simulink model "omni_interface"  (Simulink 7.0)
settings: Solver=ode1  StartTime=0.0  StopTime=inf  FixedStep=0.001  RelTol=1e-3
undefined symbols (not defined in the file): HIL
libraries: quarc_library x8, simulink x7
settings Model: Creator=colinlea  LastModifiedBy=colinlea  SimulationMode=external  ExtModeTrigDuration=10000
settings SolverCC: PositivePriorityOrder=on
settings RTWCC: SystemTargetFile=quarc_windows.tlc  TemplateMakefile=quarc_default_tmf  Description=QuaRC Win32 Target  ProcessScript=quarc_windows_make_rtw_hook
settings STFCustomTargetCC: TargetPreCompLibLocation=C:\DOCUME~1\ALLUSE~1\APPLIC~1\QuaRC\lib\2007b\windows\release  GenFloatMathFcnCalls=ANSI_C  SystemTargetFile=quarc_windows.tlc
settings GRTTargetCC: TargetPreCompLibLocation=C:\DOCUME~1\ALLUSE~1\APPLIC~1\QuaRC\lib\2007b\windows\release  CompOptLevelCompliant=off  MatFileLogging=off  ExtMode=on  ExtModeMexFile=quarc_comm

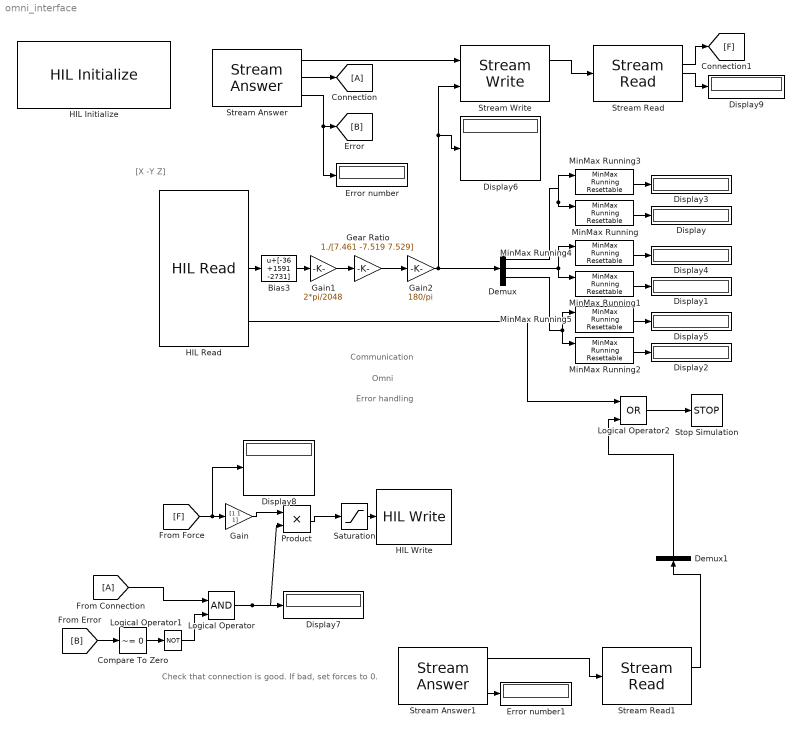
== system omni_interface ==
  note: [X -Y Z]
  note: Check that connection is good.
      | If bad, set forces to 0.
  note: Communication
  note: Omni
  note: Error handling
  Bias3 : Bias  Bias=[-36 +1591 -2731]
  Compare To Zero : simulink/Logic and Bit Operations/Compare To Zero  SystemSampleTime=-1  relop=~=  LogicOutDataTypeMode=uint8  ZeroCross=off
  Demux : Demux  Outputs=3
  Demux1 : Demux  Orientation=up  Outputs=3
  Display{,1..9} (10 alike) : Display
  Error number : Display
  Error number1 : Display
  Gain : Gain  Gain=[1 1 1]  ParameterDataType=sfix(16)  ParameterScaling=2^0  OutDataType=sfix(16)  OutScaling=2^0
  Gain1 : Gain  Gain=2*pi/2048  ParameterDataType=sfix(16)  ParameterScaling=2^0  OutDataType=sfix(16)  OutScaling=2^0
  Gain2 : Gain  Gain=180/pi  ParameterDataType=sfix(16)  ParameterScaling=2^0  OutDataType=sfix(16)  OutScaling=2^0
  Gear Ratio : Gain  Gain=1./[7.461 -7.519 7.529]  ParameterDataType=sfix(16)  ParameterScaling=2^0  OutDataType=sfix(16)  OutScaling=2^0
  HIL Initialize : quarc_library/Data Acquisition/Generic/Configuration/HIL Initialize  object_name=HIL-1  board_type=phantom_omni  board_number=0  active=on  hardware_clocks=[]  clock_modes=[]  set_clock_params_at_start=off  set_clock_params_at_switch_in=off  analog_input_channels=0:1  analog_input_maximums=10  analog_input_minimums=-10  set_analog_input_params_at_start=off  set_analog_input_params_at_switch_in=off  analog_output_channels=[]  analog_output_maximums=[]  analog_output_minimums=[]  initial_analog_outputs=[]  final_analog_outputs=[]  watchdog_analog_outputs=[]  set_analog_output_params_at_start=off  set_analog_output_params_at_switch_in=off  set_analog_outputs_at_start=off  set_analog_outputs_at_switch_in=off  set_analog_outputs_at_terminate=off  set_analog_outputs_at_switch_out=off  set_analog_outputs_on_watchdog=off  digital_input_channels=[]  digital_output_channels=[]  initial_digital_outputs=[]  final_digital_outputs=[]  watchdog_digital_outputs=[]  set_digital_outputs_at_start=off  set_digital_outputs_at_switch_in=off  set_digital_outputs_at_terminate=off  set_digital_outputs_at_switch_out=off  set_digital_outputs_on_watchdog=off  encoder_channels=0:2  quadrature=[]  encoder_filter_frequency=[]  initial_encoder_counts=0  set_encoder_params_at_start=off  set_encoder_params_at_switch_in=off  set_encoder_counts_at_start=off  set_encoder_counts_at_switch_in=off  pwm_channels=0:2  pwm_modes=[]  pwm_frequency=[]  initial_pwm_outputs=0  final_pwm_outputs=0  watchdog_pwm_outputs=[]  set_pwm_params_at_start=off  set_pwm_params_at_switch_in=off  set_pwm_outputs_at_start=on  set_pwm_outputs_at_switch_in=off  set_pwm_outputs_at_terminate=on  set_pwm_outputs_at_switch_out=off  set_pwm_outputs_on_watchdog=off  other_output_channels=[]  initial_other_outputs=[]  final_other_outputs=[]  watchdog_other_outputs=[]  set_other_outputs_at_start=off  set_other_outputs_at_switch_in=off  set_other_outputs_at_terminate=off  set_other_outputs_at_switch_out=off  set_other_outputs_on_watchdog=off
  HIL Read : quarc_library/Data Acquisition/Generic/Immediate I//O/HIL Read  object_name=HIL-1  analog_channels=[0:2]  encoder_channels=[0:2]  digital_channels=[0:1]  other_channels=[]  sample_time=qc_get_step_size  active=on  vector_output=on  data_type_mode=Inherit via back propagation  encoder_data_type=double  digital_data_type=boolean
  HIL Write : quarc_library/Data Acquisition/Generic/Immediate I//O/HIL Write  object_name=HIL-1  analog_channels=[]  pwm_channels=[0:2]  digital_channels=[]  other_channels=[]  sample_time=-1  active=off  vector_input=on
  Logical Operator : Logic  IconShape=distinctive  AllPortsSameDT=off  OutDataTypeMode=boolean
  Logical Operator1 : Logic  Operator=NOT  IconShape=distinctive  AllPortsSameDT=off  OutDataTypeMode=boolean
  Logical Operator2 : Logic  Operator=OR  Inputs=3  IconShape=distinctive  AllPortsSameDT=off  OutDataTypeMode=boolean
  MinMax Running : simulink/Math Operations/MinMax Running Resettable  SystemSampleTime=-1  Function=min  vinit=0.0
  MinMax Running1 : simulink/Math Operations/MinMax Running Resettable  SystemSampleTime=-1  Function=min  vinit=0.0
  MinMax Running2 : simulink/Math Operations/MinMax Running Resettable  SystemSampleTime=-1  Function=min  vinit=0.0
  MinMax Running3 : simulink/Math Operations/MinMax Running Resettable  SystemSampleTime=-1  Function=max  vinit=0.0
  MinMax Running4 : simulink/Math Operations/MinMax Running Resettable  SystemSampleTime=-1  Function=max  vinit=0.0
  MinMax Running5 : simulink/Math Operations/MinMax Running Resettable  SystemSampleTime=-1  Function=max  vinit=0.0
  Product : Product  OutDataType=sfix(16)  OutScaling=2^0  RndMeth=Zero
  Saturation : Saturate  UpperLimit=1  LowerLimit=-1  OutDataType=sfix(16)  OutScaling=2^0
  Stop Simulation : Stop
  Stream Answer : quarc_library/Communications/Intermediate/Stream Answer  uri_source=Internal (dialog parameter)  uri=tcpip://localhost:18000  send_buffer_size=8000  receive_buffer_size=8000  byte_order=little endian (Intel - LSB first)  sample_time=qc_get_step_size  active=off
      settings: AttributesFormatString=(%<uri>)
  Stream Answer1 : quarc_library/Communications/Intermediate/Stream Answer  uri_source=Internal (dialog parameter)  uri=tcpip://localhost:18002  send_buffer_size=8000  receive_buffer_size=8000  byte_order=little endian (Intel - LSB first)  sample_time=qc_get_step_size  active=off
      settings: AttributesFormatString=(%<uri>)
  Stream Read : quarc_library/Communications/Intermediate/Stream Read  data_type=Inherited via back propagation  num_elements=3
  Stream Read1 : quarc_library/Communications/Intermediate/Stream Read  data_type=Inherited via back propagation  num_elements=3
  Stream Write : quarc_library/Communications/Intermediate/Stream Write  optimization=Minimizing latency
  wires:
  Saturation/1 -> HIL Write/1
  MinMax Running/1 -> Display/1
  MinMax Running1/1 -> Display1/1
  MinMax Running2/1 -> Display2/1
  MinMax Running3/1 -> Display3/1
  MinMax Running4/1 -> Display4/1
  MinMax Running5/1 -> Display5/1
  Demux/1 -> MinMax Running/1, MinMax Running3/1
  Demux/2 -> MinMax Running1/1, MinMax Running4/1
  Demux/3 -> MinMax Running2/1, MinMax Running5/1
  HIL Read/2 -> Bias3/1
  Bias3/1 -> Gain1/1
  Gain1/1 -> Gear Ratio/1
  Gear Ratio/1 -> Gain2/1
  Stream Answer/1 -> Stream Write/1
  Gain2/1 -> Demux/1, Display6/1, Stream Write/2
  Gain/1 -> Product/1
  Product/1 -> Saturation/1
  Stream Answer/2 -> [A]
  Stream Answer/3 -> [B], Error number/1
  [B] -> Compare To Zero/1
  [A] -> Logical Operator/1
  Logical Operator/1 -> Product/2, Display7/1
  Stream Write/1 -> Stream Read/1
  Stream Read/2 -> [F]
  [F] -> Gain/1, Display8/1
  Stream Read/3 -> Display9/1
  Compare To Zero/1 -> Logical Operator1/1
  Logical Operator1/1 -> Logical Operator/2
  HIL Read/3 -> Logical Operator2/1
  Logical Operator2/1 -> Stop Simulation/1
  Stream Answer1/1 -> Stream Read1/1
  Stream Answer1/3 -> Error number1/1
  Stream Read1/2 -> Demux1/1
  Demux1/2 -> Logical Operator2/3
